simulink model "Control_object"  (R2022b)
settings: Solver=VariableStepAuto  StartTime=0.0  StopTime=10.0  FixedStep=0.001  RelTol=1e-3
undefined symbols (not defined in the file): i_gearbox_1, i_gearbox_2
settings Model: Creator=Maxim Kozlov  LastModifiedBy=Maxim Kozlov
settings OptimizationCC: ReuseModelBlockBuffer=on
settings ModelReferenceCC: EnableParallelModelReferenceBuilds=on

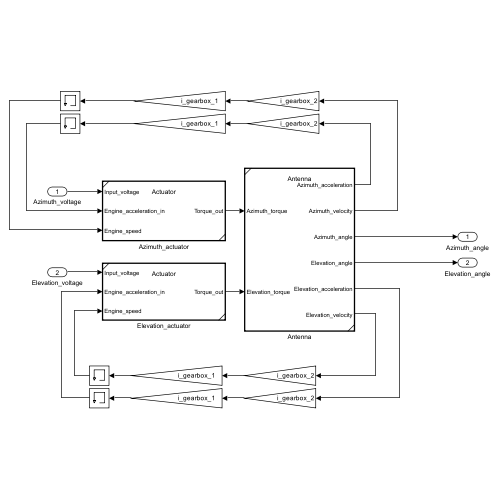
[thumbnail: Simulink's stored preview of the top-level diagram]
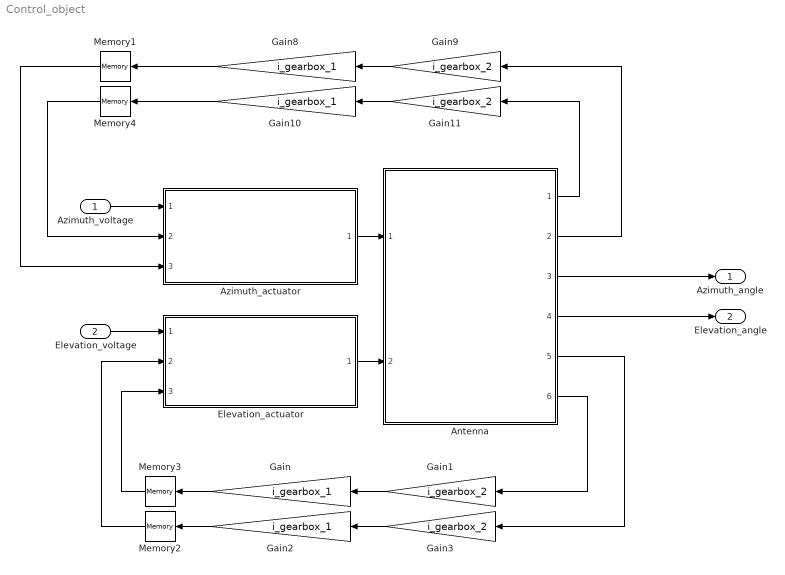
== system Control_object ==
  Azimuth_voltage : Inport
  Elevation_voltage : Inport  Port=2
  Antenna : Subsystem  TreatAsAtomicUnit=on  ReferencedSubsystem=Antenna
      settings: MinAlgLoopOccurrences=on
  Azimuth_actuator : Subsystem  TreatAsAtomicUnit=on  ReferencedSubsystem=Actuator
      settings: MinAlgLoopOccurrences=on
  Elevation_actuator : Subsystem  TreatAsAtomicUnit=on  ReferencedSubsystem=Actuator
      settings: MinAlgLoopOccurrences=on
  Gain{,2,8,10} (4 alike) : Gain  Gain=i_gearbox_1
  Gain{1,3,9,11} (4 alike) : Gain  Gain=i_gearbox_2
  Memory{1..4} (4 alike) : Memory  InheritSampleTime=on
  Azimuth_angle : Outport
  Elevation_angle : Outport  Port=2
  wires:
  Antenna/1 -> Gain11/1
  Gain8/1 -> Memory1/1
  Gain9/1 -> Gain8/1
  Elevation_voltage/1 -> Elevation_actuator/1
  Gain/1 -> Memory3/1
  Gain1/1 -> Gain/1
  Gain11/1 -> Gain10/1
  Antenna/5 -> Gain3/1
  Antenna/6 -> Gain1/1
  Elevation_actuator/1 -> Antenna/2
  Gain3/1 -> Gain2/1
  Antenna/2 -> Gain9/1
  Azimuth_actuator/1 -> Antenna/1
  Antenna/3 -> Azimuth_angle/1
  Antenna/4 -> Elevation_angle/1
  Azimuth_voltage/1 -> Azimuth_actuator/1
  Gain10/1 -> Memory4/1
  Memory1/1 -> Azimuth_actuator/3
  Gain2/1 -> Memory2/1
  Memory3/1 -> Elevation_actuator/3
  Memory2/1 -> Elevation_actuator/2
  Memory4/1 -> Azimuth_actuator/2
